simulink model "SolarPowerInverterModel"  (R2024a)
settings: Solver=ode23t  StartTime=0.0  StopTime=0.1  RelTol=1e-3
PreLoadFcn:
  | addpath(genpath('Data'));
undefined symbols (not defined in the file): Ts
libraries: nesl_utility x11, fl_lib x8, ee_lib x6, spsPWMGenerator2LevelLib x1, spsPowerLib x1, simulink x1
settings Model: Creator=callie  LastModifiedBy=callie
settings DataIOCC: InspectSignalLogs=on

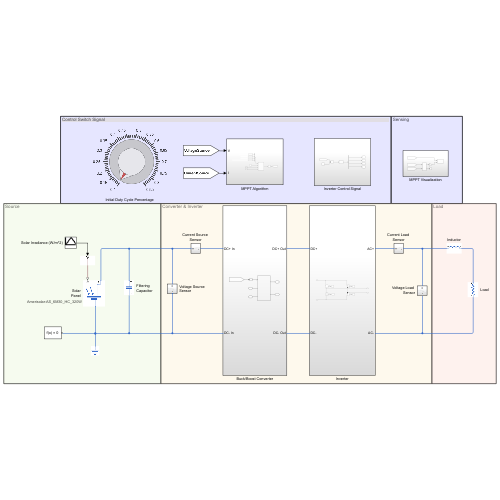
[thumbnail: Simulink's stored preview of the top-level diagram]
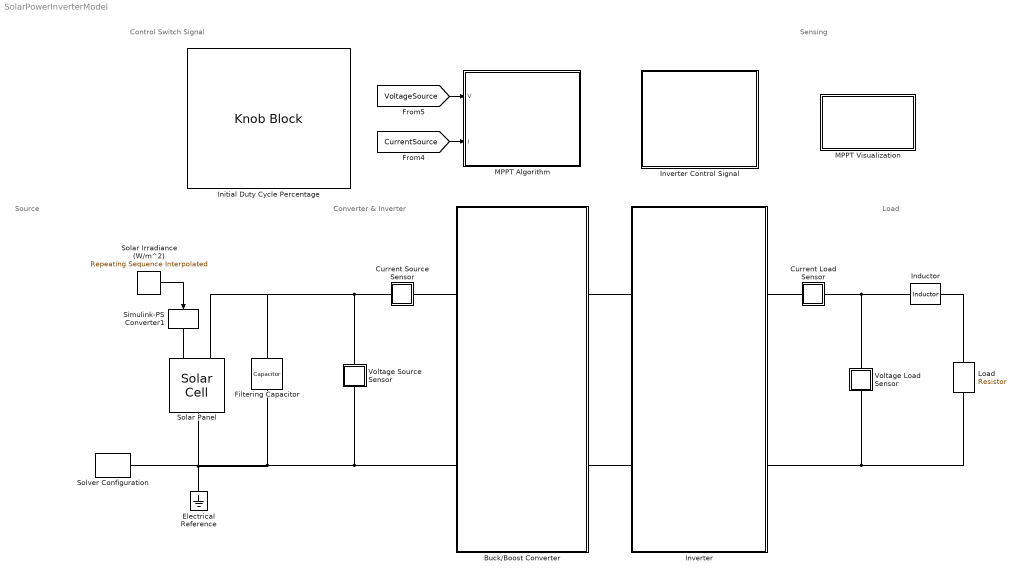
== system SolarPowerInverterModel ==
  note: Control Switch Signal
  note: Source
  note: Load
  note: Converter & Inverter
  note: Sensing
  Buck/Boost Converter : Subsystem
  Current Load Sensor : Subsystem
  Current Source Sensor : Subsystem
  Electrical Reference : fl_lib/Electrical/Electrical Elements/Electrical Reference
  Filtering Capacitor : fl_lib/Electrical/Electrical Elements/Capacitor  c=5e-3 F  r=1e-6 Ohm  g=0 1/Ohm  i_specify=off  i_priority=None  i=0 A  i_nominal_specify=off  i_nominal_value=1  i_nominal_unit=A  v_specify=off  v_priority=None  v=0 V  v_nominal_specify=off  v_nominal_value=1  v_nominal_unit=V  vc_specify=off  vc_priority=High  vc=0 V  vc_nominal_specify=off  vc_nominal_value=1  vc_nominal_unit=V
  Inductor : fl_lib/Electrical/Electrical Elements/Inductor  l=2e-3 H  r=0 Ohm  g=0 1/Ohm  i_specify=off  i_priority=None  i=0 A  i_nominal_specify=off  i_nominal_value=1  i_nominal_unit=A  v_specify=off  v_priority=None  v=0 V  v_nominal_specify=off  v_nominal_value=1  v_nominal_unit=V  i_L_specify=off  i_L_priority=High  i_L=0 A  i_L_nominal_specify=off  i_L_nominal_value=1  i_L_nominal_unit=A
  Initial Duty Cycle Percentage : KnobBlock  LabelPosition=Hide  ScaleMin=0.1  ScaleMax=0.85  TickInterval=0.05
  Inverter : Subsystem
  Inverter Control Signal : Subsystem
  Load : fl_lib/Electrical/Electrical Elements/Resistor  R=25 Ohm  i_specify=off  i_priority=High  i=0 A  i_nominal_specify=off  i_nominal_value=1  i_nominal_unit=A  v_specify=off  v_priority=High  v=0 V  v_nominal_specify=off  v_nominal_value=1  v_nominal_unit=V
  MPPT Algorithm : Subsystem
  MPPT Visualization : Subsystem
  Simulink-PS Converter1 : nesl_utility/Simulink-PS Converter  PhysicalDomain=network_engine_domain  SubClassName=ps_input  LeftPortType=input  RightPortType=output  PseudoPeriodic=off  Frequencies=[]  NoiseDistribution=none  NoiseParameters=[]  Unit=W/m^2  AffineConversion=off  FilteringAndDerivatives=zero  SimscapeFilterOrder=1  InputFilterTimeConstant=0.001  UdotUserProvided=1
  Solar Panel : ee_lib/Sources/Solar Cell  Tag={'toolbox/physmod/elec/library/m/ee_lib_parts';'Sources/Solar_Cell/Amerisolar/AS_6M30_HC_320W.xml'}  prm=3  Isc=10.14 A  Voc=0.67 V  Is=3.24823447983853e-07 A  Is2=9.37081970792037e-10 A  Iph=10.140005507508 A  Ir0=1000 W/m^2  ec=1.51118472243322  N2=2.60259908345858  Rs=1.94548269975201e-05 Ohm  Rp=682.95993142779 Ohm  N_series=60  N_parallel=1  TIPH1=0.000499942933005141 1/K  EG=1.12 eV  TXIS1=4.23641510120988  TXIS2=16.2689137700667  TRS1=0.243341028305912  TRP1=0 % Parameter not set  Tmeas=25 degC  TFIXED=30 degC  thermal_mass=100 % Parameter not set J/K  initial_temperature=25 degC
      settings: AttributesFormatString=Amerisolar:AS_6M30_HC_320W
  Solar Irradiance (W/m^2) : simulink/Sources/Repeating Sequence Interpolated  OutValues=[0 0 1 1 2 2 3 3 4 4 5 5 6 6 5 5 4 4 3 3 2 2 1 1]*200  TimeValues=[0 1 2 3 4 5 6 7 8 9 10 11 12 13 14 15 16 17 18 19 20 21 22 23]/230  LookUpMeth=Interpolation-Use End Values  tsamp=0.001  OutMin=[]  OutMax=[]  OutDataTypeStr=double  OutputDataTypeScalingMode=double  OutDataType=fixdt(0,8)  OutScaling=2^-10
  Solver Configuration : nesl_utility/Solver Configuration  PhysicalDomain=network_engine_domain  SubClassName=solver  LeftPortType=input  RightPortType=generic  Tones=[]  Harmonics=[]  SimulateNoise=off  Profile=off  UseLocalSampling=off  EnableSwitchedLinearOptims=on  FrequencyDomain=off  UseCCode=off  RelTol=0.001  AbsTol=0.001  MinStep=1e-09  ToWorkspace=off  RevertToSquareIcSolve=off  NumHomotopyIterations=100  PhasorMode=off  PhasorModeNumHarmonics=1  ConsistencySolver=NEWTON_XTOL_AFTER_FTOL  IndexReductionMethod=DerivativeReplacement  DoDC=off  ResidualTolerance=1e-09  ConsistencyTolSource=GLOBAL  ConsistencyAbsTol=0.001  ConsistencyRelTol=0.001  ConsistencyTolFactor=0.001  UseLocalSolver=on  LocalSolverChoice=NE_BACKWARD_EULER_ADVANCER  ResolveIndetEquations=on  FunctionEvalNumThread=1  LocalSolverSampleTime=1e-6  DoFixedCost=on  MaxNonlinIter=3  MaxModeIter=2  ComputeImpulses=off  ImpulseIterations=2  LinearAlgebra=auto  LinearAlgebraNumThread=0  EquationFormulation=NE_TIME_EF  DelaysMemoryBudget=1024  AutomaticFiltering=on  FilteringTimeConstant=0.001  PartitionStorageMethod=AS_NEEDED  PartitionMemoryBudget=1024  PartitionMethod=ROBUST  MultibodyUseLocalSolver=off  MultibodyLocalSolverChoice=ODE1  MultibodyLocalSolverSampleTime=0.001
  Voltage Load Sensor : Subsystem
  Voltage Source Sensor : Subsystem
  wires:
  [CurrentSource] -> MPPT Algorithm/2(I)
  [VoltageSource] -> MPPT Algorithm/1(V)
  Solar Irradiance (W/m^2)/1 -> Simulink-PS Converter1/1
  connections:
  Buck/Boost Converter/LConn2 -- Voltage Source Sensor/RConn1 -- Electrical Reference/LConn1 -- Solver Configuration/RConn1 -- Solar Panel/RConn1 -- Filtering Capacitor/RConn1
  Load/RConn1 -- Voltage Load Sensor/RConn1 -- Inverter/RConn2
  Current Source Sensor/LConn1 -- Filtering Capacitor/LConn1 -- Solar Panel/LConn2 -- Voltage Source Sensor/LConn1
  Buck/Boost Converter/LConn1 -- Current Source Sensor/RConn1
  Buck/Boost Converter/RConn1 -- Inverter/LConn1
  Buck/Boost Converter/RConn2 -- Inverter/LConn2
  Current Load Sensor/LConn1 -- Inverter/RConn1
  Simulink-PS Converter1/RConn1 -- Solar Panel/LConn1
  Voltage Load Sensor/LConn1 -- Inductor/LConn1 -- Current Load Sensor/RConn1
  Inductor/RConn1 -- Load/LConn1

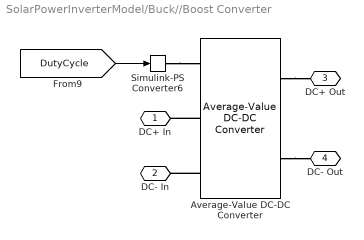
== system SolarPowerInverterModel/Buck//Boost Converter ==
  Average-Value DC-DC Converter : ee_lib/Semiconductors & Converters/Converters/Average-Value DC-DC Converter  control_option=ee.enum.converters.controlinput.dutycycle  converter_type=ee.enum.converters.dcdctype.buckboost  efficiency_option=ee.enum.converters.efficiency.constant  efficiency_fixed=100  i_vec=[0, 2, 5] A  efficiency_vec=[90, 95, 98]
      settings: InternalSimscapePortConfiguration="{\"Bottom\":[],\"Left\":[{\"id\":\"DutyCycle\",\"label\":\"DutyCycle\",\"type\":\"input\"},{\"id\":\"p1\",\"label\":\"1+\",\"type\":\"foundation.electrical.electrical\"},{\"id\":\"n1\",\"label\":\"1-\",\"type\":\"foundation.electrical.electrical\"}],\"Right\":[{\"id\":\"p2\",\"label\":\"2+\",\"type\":\"foundation.electrical.electrical\"},{\"id\":\"n2\",\"label\":\"2-\",\"type\":\"foundation.electrical.electrical\"}],\"Top\":[]}"
  Simulink-PS Converter6 : nesl_utility/Simulink-PS Converter  PhysicalDomain=network_engine_domain  SubClassName=ps_input  LeftPortType=input  RightPortType=output  PseudoPeriodic=off  Frequencies=[]  NoiseDistribution=none  NoiseParameters=[]  Unit=1  AffineConversion=off  FilteringAndDerivatives=provide  SimscapeFilterOrder=1  InputFilterTimeConstant=0.001  UdotUserProvided=0
  DC+ In : PMIOPort  Side=Left
  DC- In : PMIOPort  Port=2  Side=Left
  DC+ Out : PMIOPort  Port=3  Side=Right
  DC- Out : PMIOPort  Port=4  Side=Right
  wires:
  [DutyCycle] -> Simulink-PS Converter6/1
  connections:
  Average-Value DC-DC Converter/RConn1 -- DC+ Out/RConn1
  Simulink-PS Converter6/RConn1 -- Average-Value DC-DC Converter/LConn1
  Average-Value DC-DC Converter/LConn3 -- DC- In/RConn1
  Average-Value DC-DC Converter/RConn2 -- DC- Out/RConn1
  Average-Value DC-DC Converter/LConn2 -- DC+ In/RConn1

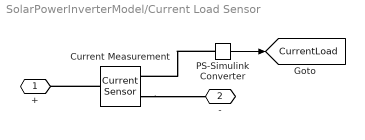
== system SolarPowerInverterModel/Current Load Sensor ==
  Current Measurement : fl_lib/Electrical/Electrical Sensors/Current Sensor
  PS-Simulink Converter : nesl_utility/PS-Simulink Converter  PhysicalDomain=network_engine_domain  SubClassName=ps_output  LeftPortType=input  RightPortType=output  PseudoPeriodic=off  Frequencies=[]  VectorFormat=1-D array  Unit=inherit  AffineConversion=off
  + : PMIOPort  Side=Left
  - : PMIOPort  Port=2  Side=Right
  tag scope: CurrentLoad=global
  wires:
  PS-Simulink Converter/1 -> [CurrentLoad]
  connections:
  Current Measurement/RConn2 -- -/RConn1
  Current Measurement/LConn1 -- +/RConn1
  PS-Simulink Converter/LConn1 -- Current Measurement/RConn1

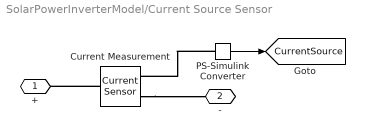
== system SolarPowerInverterModel/Current Source Sensor ==
  Current Measurement : fl_lib/Electrical/Electrical Sensors/Current Sensor
  PS-Simulink Converter : nesl_utility/PS-Simulink Converter  PhysicalDomain=network_engine_domain  SubClassName=ps_output  LeftPortType=input  RightPortType=output  PseudoPeriodic=off  Frequencies=[]  VectorFormat=1-D array  Unit=inherit  AffineConversion=off
  + : PMIOPort  Side=Left
  - : PMIOPort  Port=2  Side=Right
  tag scope: CurrentSource=global
  wires:
  PS-Simulink Converter/1 -> [CurrentSource]
  connections:
  PS-Simulink Converter/LConn1 -- Current Measurement/RConn1
  Current Measurement/LConn1 -- +/RConn1
  Current Measurement/RConn2 -- -/RConn1

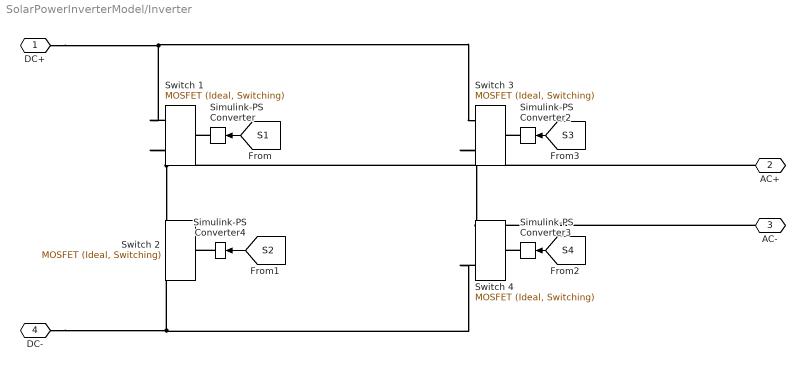
== system SolarPowerInverterModel/Inverter ==
  Simulink-PS Converter{,2..4} (4 alike) : nesl_utility/Simulink-PS Converter  PhysicalDomain=network_engine_domain  SubClassName=ps_input  LeftPortType=input  RightPortType=output  PseudoPeriodic=off  Frequencies=[]  NoiseDistribution=none  NoiseParameters=[]  Unit=1  AffineConversion=off  FilteringAndDerivatives=provide  SimscapeFilterOrder=1  InputFilterTimeConstant=0.001  UdotUserProvided=0
  Switch {1..4} (4 alike) : ee_lib/Semiconductors & Converters/MOSFET (Ideal, Switching)  port_option=ee.enum.controlport.ps  Rds=1e-3 Ohm  Goff=1e-6 1/Ohm  Vth=0.1 V  diode_param=ee.enum.semiconductors.protectionDiode.nodynamics  diode_Vf=0.6 V  diode_Ron=1e-3 Ohm  diode_Goff=1e-5 1/Ohm  diode_C=50e-9 F  diode_iRM=-235 A  diode_iF=300 A  diode_idot=-50 A/us  diode_trr_param=ee.enum.converters.diodeReverseParam.trr_factor  diode_trr_factor=3  diode_trr=15 us  diode_Qrr=1500 s*uA  ids_specify=off  ids_priority=None  ids=0 A  ids_nominal_specify=off  ids_nominal_value=1  ids_nominal_unit=A  vds_specify=off  vds_priority=None  vds=0 V  vds_nominal_specify=off  vds_nominal_value=1  vds_nominal_unit=V  vgs_specify=off  vgs_priority=None  vgs=0 V  vgs_nominal_specify=off  vgs_nominal_value=1  vgs_nominal_unit=V  thermal_loss_option=ee.enum.converters.thermalLossOption.constantvalues  Von_data=[0, 1.8, 3.2, 6, 10, 16; 0, 2, 5.5, 9.5, 15, 25] V  Tj=[298.15, 448.15] K  Iout_data=[0, 20, 40, 60, 80, 100] A  Eon_data=[0, 55.04, 124.57, 235.53, 362.12; 0, 71.25, 161.25, 304.88, 468.75] * 1e-6 J  Eoff_data=[0, 18, 30, 56.1, 76.5; 0, 22.5, 37.5, 70.13, 95.63] * 1e-6 J  Eon_data_3D=[zeros(2, 5, 3)] J  Eoff_data_3D=[zeros(2, 5, 3)] J  Tj_loss=[298.15, 448.15] K  Iout_data_loss=[0, 10, 20, 30, 40] A  tabulateWithVds=false  Vds_loss=[0, 150, 300] V  Eon_scalar=22.86e-3 J  Eoff_scalar=17.14e-3 J  Voff=300 V  Iout_scalar=600 A  useCurrentFromPreviousCycle=false  useVoltageFromPreviousCycle=false  diodeModelType=ee.enum.converters.diodeModelType.pwl  diodeTableType=ee.enum.diode.tableType.IfMat  diode_ReverseIVType=ee.enum.diode.diodeReverseIV.constant  diode_IfMat=[.07, .12, .19, 1.75, 4.24, 7.32, 11.2; .16, .3, .72, 2.14, 4.02, 6.35, 9.12] A  diode_VfMat=[.9, 1.15, 1.25, 1.5, 1.75, 2.17, 2.6, 2.85; .58, .68, .75, 1.1, 1.38, 1.77, 2.27, 2.7] V  diode_TjVec=[25, 125] degC  diode_VfVec=[.5, .7, .9, 1.3, 1.7, 2.1, 2.5] V  diode_IfVec=[.1, .2, .5, 1, 2, 4, 7, 10] A  diode_IrMat=[1e-06, 2e-06, 5e-06, 1e-05, 2.5e-05, 5e-05, .0001; 2e-06, 5e-06, 1e-05, 4e-05, 8e-05, .0002, .0005] A  diode_VrMat=[10, 100, 200, 250, 300, 325, 350; 10, 70, 160, 220, 270, 300, 320] V  diode_VrVec=[10, 20, 40, 50, 70, 80, 100] V  diode_IrVec=[1e-06, 2e-06, 5e-06, 1e-05, 2e-05, 5e-05, .0001] A  diode_Vr=-600 V  diode_Ls=150 nH  diode_Erec=0.03 J  diode_rec_loss_model=ee.enum.diode.reverseRecoveryModel.fixed  diode_ErecVal=0 J  diode_scaleWithIandV=true  diode_ErecMat=zeros(2, 3) J  diode_TjrecVec=[298.15, 398.15] K  diode_IfrecVec=[.1, 1, 10] A  diode_IrecVal=10 A  diode_VrecVal=10 V  diode_tFilter=1 / 1000 / 100 s  thermal_network_parameterization=ee.enum.thermalNetworkTopology.external  Rth=[.03, .2] K/W  Rth_Cauer=[.03, .1, .2] K/W  Rth_Foster=[.03, .2] K/W  thermal_mass_parameterization=ee.enum.thermalNetwork.timeconstant  thermal_mass=[3, 25] J/K  thermal_mass_Cauer=[3, 10, 25] J/K  thermal_mass_Foster=[33, 50] J/K  thermal_time_constant=[.1, 5] s  thermal_time_constant_Cauer=[.1, 1, 5] s  thermal_time_constant_Foster=[1, 10] s  thermal_mass_initial_temperatures=[25, 25] degC  thermal_mass_initial_temperatures_Cauer=[25, 25, 25] degC  junction_thermal_mass=0.1 J/K  Tvec_initial_Foster=[25, 25, 25, 25] degC  no_thermal_network=0  junction_temperature_specify=off  junction_temperature_priority=None  junction_temperature=25 degC  junction_temperature_nominal_specify=off  junction_temperature_nominal_value=1  junction_temperature_nominal_unit=degC  Qj_specify=off  Qj_priority=None  Qj=0 W  Qj_nominal_specify=off  Qj_nominal_value=1  Qj_nominal_unit=W  accumulatedSwitchingLosses_specify=off  accumulatedSwitchingLosses_priority=None  accumulatedSwitchingLosses=0 J
  DC+ : PMIOPort  Side=Left
  AC+ : PMIOPort  Port=2  Side=Right
  AC- : PMIOPort  Port=3  Side=Right
  DC- : PMIOPort  Port=4  Side=Left
  wires:
  [S2] -> Simulink-PS Converter4/1
  [S3] -> Simulink-PS Converter2/1
  [S1] -> Simulink-PS Converter/1
  [S4] -> Simulink-PS Converter3/1
  connections:
  Switch 1/RConn1 -- Switch 3/RConn1 -- DC+/RConn1
  Simulink-PS Converter2/RConn1 -- Switch 3/LConn1
  Switch 3/RConn2 -- AC-/RConn1 -- Switch 4/RConn1
  Switch 1/RConn2 -- AC+/RConn1 -- Switch 2/RConn1
  Switch 4/RConn2 -- DC-/RConn1 -- Switch 2/RConn2
  Simulink-PS Converter/RConn1 -- Switch 1/LConn1
  Simulink-PS Converter4/RConn1 -- Switch 2/LConn1
  Simulink-PS Converter3/RConn1 -- Switch 4/LConn1

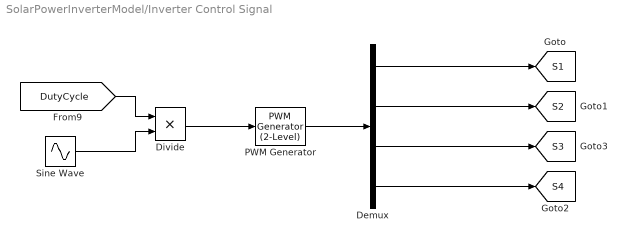
== system SolarPowerInverterModel/Inverter Control Signal ==
  Demux : Demux
  Divide : Product  Inputs=**
  PWM Generator : spsPWMGenerator2LevelLib/PWM Generator (2-Level)  ModulatorType=Single-phase full-bridge (4 pulses)  ModulatorMode=Unsynchronized  Fc=10000  Pc=90  nF=27  MinMax="[ -1  1 ]"  SamplingTechnique=Natural  ModulatingSignals=off  m=0.8  Freq=60  Phase=0  Ts=0  ShowCarrierOutport=off
  Sine Wave : Sin  Frequency=60*2*pi  SampleTime=0
  tag scope: S1=global, S2=global, S3=global, S4=global
  wires:
  Demux/2 -> [S2]
  Demux/1 -> [S1]
  Demux/3 -> [S3]
  Demux/4 -> [S4]
  PWM Generator/1 -> Demux/1
  [DutyCycle] -> Divide/1
  Divide/1 -> PWM Generator/1
  Sine Wave/1 -> Divide/2

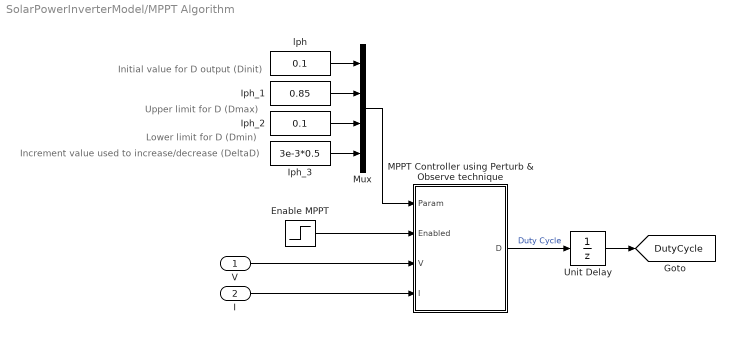
== system SolarPowerInverterModel/MPPT Algorithm ==
  note: Initial value for D output (Dinit)
  note: Increment value used to increase/decrease (DeltaD)
  note: Upper limit for D (Dmax)
  note: Lower limit for D (Dmin)
  V : Inport
  I : Inport  Port=2
  Enable MPPT : Step  Time=0.01  SampleTime=0
  Iph_1 : Constant  Value=0.85
  Iph_2 : Constant  Value=0.1
  Iph_3 : Constant  Value=3e-3*0.5
  "MPPT Controller using Perturb & Observe technique " : MATLAB Function  SystemSampleTime=Ts
  Mux : Mux
  Unit Delay : UnitDelay  InitialCondition=0.5  SampleTime=-1  HasFrameUpgradeWarning=on
  lph : Constant  Value=0.1
  tag scope: DutyCycle=global
  wires:
  V/1 -> "MPPT Controller using Perturb & Observe technique "/3(V)
  Mux/1 -> "MPPT Controller using Perturb & Observe technique "/1(Param)
  Iph_1/1 -> Mux/2
  lph/1 -> Mux/1
  Iph_2/1 -> Mux/3
  "MPPT Controller using Perturb & Observe technique "/1(D) -> Unit Delay/1  "Duty Cycle"
  Iph_3/1 -> Mux/4
  Enable MPPT/1 -> "MPPT Controller using Perturb & Observe technique "/2(Enabled)
  I/1 -> "MPPT Controller using Perturb & Observe technique "/4(I)
  Unit Delay/1 -> [DutyCycle]

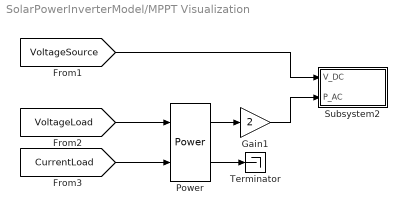
== system SolarPowerInverterModel/MPPT Visualization ==
  Gain1 : Gain  Gain=2
  Power : spsPowerLib/Power  Freq=60  Vinit=[1, 0]  Iinit=[1, 0]  Ts=0
  Subsystem2 : Subsystem
      mask Display: disp('Visualize\nOperation')
  Terminator : Terminator
  wires:
  [VoltageLoad] -> Power/1
  [VoltageSource] -> Subsystem2/1(V_DC)
  Power/1 -> Gain1/1
  [CurrentLoad] -> Power/2
  Gain1/1 -> Subsystem2/2(P_AC)
  Power/2 -> Terminator/1

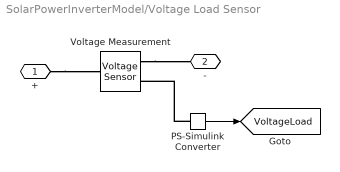
== system SolarPowerInverterModel/Voltage Load Sensor ==
  PS-Simulink Converter : nesl_utility/PS-Simulink Converter  PhysicalDomain=network_engine_domain  SubClassName=ps_output  LeftPortType=input  RightPortType=output  PseudoPeriodic=off  Frequencies=[]  VectorFormat=1-D array  Unit=inherit  AffineConversion=off
  Voltage Measurement : fl_lib/Electrical/Electrical Sensors/Voltage Sensor
  + : PMIOPort  Side=Left
  - : PMIOPort  Port=2  Side=Right
  tag scope: VoltageLoad=global
  wires:
  PS-Simulink Converter/1 -> [VoltageLoad]
  connections:
  Voltage Measurement/RConn2 -- -/RConn1
  +/RConn1 -- Voltage Measurement/LConn1
  PS-Simulink Converter/LConn1 -- Voltage Measurement/RConn1

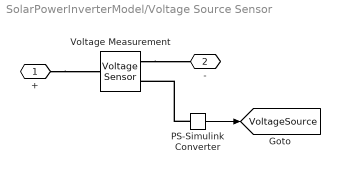
== system SolarPowerInverterModel/Voltage Source Sensor ==
  PS-Simulink Converter : nesl_utility/PS-Simulink Converter  PhysicalDomain=network_engine_domain  SubClassName=ps_output  LeftPortType=input  RightPortType=output  PseudoPeriodic=off  Frequencies=[]  VectorFormat=1-D array  Unit=inherit  AffineConversion=off
  Voltage Measurement : fl_lib/Electrical/Electrical Sensors/Voltage Sensor
  + : PMIOPort  Side=Left
  - : PMIOPort  Port=2  Side=Right
  tag scope: VoltageSource=global
  wires:
  PS-Simulink Converter/1 -> [VoltageSource]
  connections:
  PS-Simulink Converter/LConn1 -- Voltage Measurement/RConn1
  +/RConn1 -- Voltage Measurement/LConn1
  Voltage Measurement/RConn2 -- -/RConn1

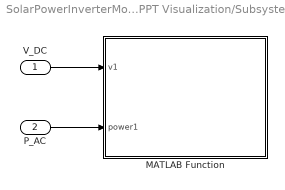
== system SolarPowerInverterModel/MPPT Visualization/Subsystem2 ==
  V_DC : Inport
  P_AC : Inport  Port=2
  MATLAB Function : MATLAB Function  TreatAsAtomicUnit=on  SystemSampleTime=Tanim  mask(Machine Rotor Animation){Tanim=0.0004}
      mask prompts: Tanim "Animation Rate [s]"
      mask help: This block animates permanent magnet inside a stator. The "thetaRotor" input is the angle of the rotor. The "phase" parameter must be defined in the workspace and selects the energized coil in the stator.
  wires:
  V_DC/1 -> MATLAB Function/1(v1)
  P_AC/1 -> MATLAB Function/2(power1)

== matlab function SolarPowerInverterModel/MPPT Visualization/Subsystem2/MATLAB Function ==
  data: v1 input; power1 input
function powerTracking(v1,power1)

% Copyright 2022, The MathWorks, Inc.

persistent hf hg1

if isempty(hf)
    
    figure(1); clf(1); hold on;
    
    [hf,hg1] = plotBackground(v1,power1);

    drawnow
    
else
    
    updateAnimation(hg1,v1,power1);

    drawnow

end

end


function [hf,hg1] = plotBackground(speed1,power1)

hf = figure(1);hold on;box on
set(hf,'Color','w')


y = load('solarPanel1LUT.mat');

set(hf,'Color',[1 1 1])
plot(y.vVec,y.powerMat,'LineWidth',1,'Color','b');
temp_ylim = get(gca,'YLim');
set(gca,'YLim',[0 temp_ylim(2)]); % Only show positive results
grid on
title('Solar Cell Power Curves at 30 degC and Varying Irradiance');
xlabel('Output Voltage (V)')
ylabel('Output Power (W)')

% maximum power curve

hold on,plot(y.solarPanel1.voltageTable(2:7),y.solarPanel1.powerTable(2:7),'r')
irradianceVec = 0:200:1200;

nn = {
    'Ir = 200 W/m2'
    'Ir = 400 W/m2'
    'Ir = 600 W/m2'
    'Ir = 800 W/m2'
    'Ir = 1000 W/m2'
    'Ir = 1200 W/m2'
    };

for x = 2:7

    text(y.solarPanel1.voltageTable(x)+2.5,y.solarPanel1.powerTable(x),nn{x-1})


end

hg1 = plot(speed1,power1,'o');
set(hg1,'Color','b')
set(hg1,'MarkerFaceColor','g')
set(hg1,'MarkerSize',10)

end


function  updateAnimation(hg1,speed1,power1)

set(hg1,'XData',speed1)
set(hg1,'YData',power1)



end

== matlab function SolarPowerInverterModel/MPPT Algorithm/MPPT Controller using Perturb & Observe technique  ==
  settings: updateMethod=DISCRETE  sampleTime=1e-3
  data: Param input; Enabled input; V input; I input; D output
function D  = PandO(Param, Enabled, V, I)

% MPPT controller based on the Perturb & Observe algorithm.

% D output = Duty cycle of the boost converter (value between 0 and 1)
%
% Enabled input = 1 to enable the MPPT controller
% V input = PV array terminal voltage (V)
% I input = PV array current (A)
%
% Param input:
Dinit = Param(1);  %Initial value for D output
Dmax = Param(2);   %Maximum value for D
Dmin = Param(3);   %Minimum value for D
deltaD = Param(4); %Increment value used to increase/decrease the duty cycle D
% ( increasing D = decreasing Vref )
%  

persistent Vold Pold Dold;

dataType = 'double';

if isempty(Vold)
    Vold=0;
    Pold=0;
    Dold=Dinit;
end
P= V*I;
dV= V - Vold;
dP= P - Pold;

 if dP ~= 0 & Enabled ~=0
%     if dP>1e-9  & dP<-1e-9 & Enabled ~=0
    if dP < 0
        if dV < 0
            D = Dold - deltaD;
        else
            D = Dold + deltaD;
        end
    else
        if dV < 0
            D = Dold + deltaD;
        else
            D = Dold - deltaD;
        end    
    end
else D=Dold;
end

if D >= Dmax | D<= Dmin
    D=Dold;
end

Dold=D;
Vold=V;
Pold=P;
